simulink model "Project_P40_1"  (R2017b)
settings: Solver=VariableStepAuto  StartTime=0.0  StopTime=10.0  RelTol=1e-3
settings Model: Creator=Administrator  LastModifiedBy=Administrator

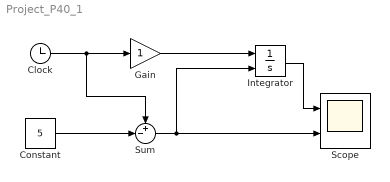
== system Project_P40_1 ==
  Clock : Clock
  Constant : Constant  Value=5
  Gain : Gain
  Integrator : Integrator  ExternalReset=rising
  Scope : Scope  NumInputPorts=2
  Sum : Sum  Inputs=+-|
  wires:
  Clock/1 -> Sum/1, Gain/1
  Gain/1 -> Integrator/1
  Integrator/1 -> Scope/1
  Constant/1 -> Sum/2
  Sum/1 -> Integrator/2, Scope/2
